simulink model "xaui_loop_delay"  (Simulink 7.0)
settings: Solver=ode45  StartTime=0.0  StopTime=100  RelTol=1e-3
undefined symbols (not defined in the file): iBOB
libraries: xbsIndex_r4 x16, xps_library x11, isi_correlator_lib x4
settings Model: Creator=wjm  LastModifiedBy=wjm

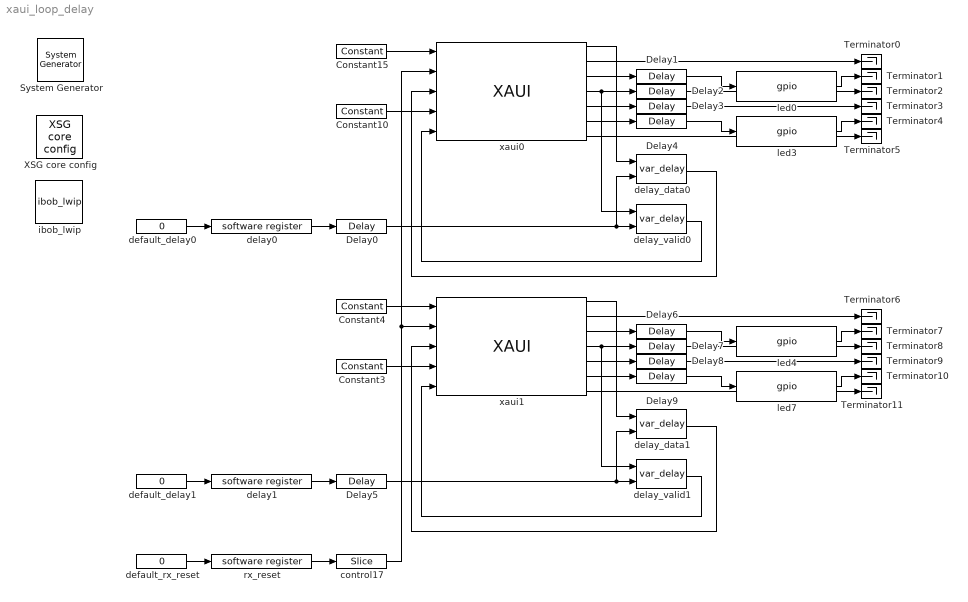
== system xaui_loop_delay ==
  " System Generator" : xbsIndex_r4/ System Generator  Tag=genX  SystemSampleTime=-1  xilinxfamily=virtex2p  part=xc2vp50  speed=-7  package=ff1152  synthesis_tool=XST  clock_wrapper=Clock Enables  directory=./xaui_loop_delay/sysgen  testbench=off  simulink_period=1  sysclk_period=5  dcm_input_clock_period=100  incr_netlist=off  trim_vbits=Everywhere in SubSystem  dbl_ovrd=According to Block Masks  core_generation=According to Block Masks  run_coregen=off  deprecated_control=off  eval_field=0  block_type=sysgen
      settings: block_version=10.1.1
  Constant10 : xbsIndex_r4/Constant  arith_type=Unsigned  const=0  n_bits=8  bin_pt=0  explicit_period=on  period=1  equ=P=C  opselect=C  inp2=PCIN>>17  opr=+  inp1=P  carry=CIN  dbl_ovrd=off  block_type=constant
      settings: block_version=10.1.1
  Constant15 : xbsIndex_r4/Constant  arith_type=Boolean  const=1  n_bits=1  bin_pt=0  explicit_period=on  period=1  equ=P=C  opselect=C  inp2=PCIN>>17  opr=+  inp1=P  carry=CIN  dbl_ovrd=off  block_type=constant
      settings: block_version=10.1.1
  Constant3 : xbsIndex_r4/Constant  arith_type=Unsigned  const=0  n_bits=8  bin_pt=0  explicit_period=on  period=1  equ=P=C  opselect=C  inp2=PCIN>>17  opr=+  inp1=P  carry=CIN  dbl_ovrd=off  block_type=constant
      settings: block_version=10.1.1
  Constant4 : xbsIndex_r4/Constant  arith_type=Boolean  const=1  n_bits=1  bin_pt=0  explicit_period=on  period=1  equ=P=C  opselect=C  inp2=PCIN>>17  opr=+  inp1=P  carry=CIN  dbl_ovrd=off  block_type=constant
      settings: block_version=10.1.1
  Delay{0..9} (10 alike) : xbsIndex_r4/Delay  en=off  latency=1  dbl_ovrd=off  reg_retiming=off  block_type=delay
  Terminator{0..11} (12 alike) : Terminator
  XSG core config : xps_library/XSG core config  Tag=xps:xsg  SystemSampleTime=-1  hw_sys=iBOB  ibob_linux=off  clk_src=sys_clk2x  iBOB_clk_src=sys_clk2x  BEE2_ctrl_clk_src=sys_clk  BEE2_usr_clk_src=sys_clk  ROACH_clk_src=adc0_clk  CORR_clk_src=sys_clk  gpio_clk_io_group=iBOB:sma  gpio_clk_bit_index=0  clk_rate=200  sample_period=1  synthesis_tool=XST  mpc_type=powerpc405
  control17 : xbsIndex_r4/Slice  nbits=1  boolean_output=on  mode=Lower Bit Location + Width  bit1=0  base1=MSB of Input  bit0=0  base0=LSB of Input  dbl_ovrd=off  block_type=slice
      settings: infoedit="Extracts a given range of bits from each input sample and presents it at the output.  The output type is ordinarily unsigned with binary point at zero, but can be Boolean when the slice is one bit wide.<P><P>Hardware notes: In hardware this block costs nothing."  block_version=10.1.3
  default_delay0 : Constant  Value=0  OutDataType=sfix(16)  OutScaling=2^0  SampleTime=1
  default_delay1 : Constant  Value=0  OutDataType=sfix(16)  OutScaling=2^0  SampleTime=1
  default_rx_reset : Constant  Value=0  OutDataType=sfix(16)  OutScaling=2^0  SampleTime=1
  delay0 : xps_library/software register  Tag=xps:sw_reg  SystemSampleTime=-1  io_dir=From Processor  arith_type=Unsigned  bitwidth=32  bin_pt=0  sample_period=1  gw_name=xaui_loop_delay_delay0_user_data_out
      link override xaui_loop_delay_delay0_user_data_out: arith_type=Unsigned  n_bits=32  bin_pt=0  period=1
  delay1 : xps_library/software register  Tag=xps:sw_reg  SystemSampleTime=-1  io_dir=From Processor  arith_type=Unsigned  bitwidth=32  bin_pt=0  sample_period=1  gw_name=xaui_loop_delay_delay1_user_data_out
      link override xaui_loop_delay_delay1_user_data_out: arith_type=Unsigned  n_bits=32  bin_pt=0  period=1
  delay_data0 : isi_correlator_lib/var_delay  SystemSampleTime=-1
  delay_data1 : isi_correlator_lib/var_delay  SystemSampleTime=-1
  delay_valid0 : isi_correlator_lib/var_delay  SystemSampleTime=-1
  delay_valid1 : isi_correlator_lib/var_delay  SystemSampleTime=-1
  ibob_lwip : xps_library/ibob_lwip  SystemSampleTime=-1
      link override macbits/convert: arith_type=Unsigned  n_bits=32  bin_pt=0
      link override machdr/xaui_loop_delay_ibob_lwip_machdr_gateway: arith_type=Unsigned  n_bits=20  bin_pt=0  period=sample_period
  led0 : xps_library/gpio  Tag=xps:gpio  SystemSampleTime=-1  io_group=iBOB:led  io_dir=out  arith_type=Boolean  bitwidth=1  bin_pt=0  bit_index=1  sample_period=1  use_single_ended=off  use_ddr=off  reg_iob=on  reg_clk_phase=0  termination=None
      link override convert: arith_type=Boolean  n_bits=1  bin_pt=0
  led3 : xps_library/gpio  Tag=xps:gpio  SystemSampleTime=-1  io_group=iBOB:led  io_dir=out  arith_type=Boolean  bitwidth=1  bin_pt=0  bit_index=2  sample_period=1  use_single_ended=off  use_ddr=off  reg_iob=on  reg_clk_phase=0  termination=None
      link override convert: arith_type=Boolean  n_bits=1  bin_pt=0
  led4 : xps_library/gpio  Tag=xps:gpio  SystemSampleTime=-1  io_group=iBOB:led  io_dir=out  arith_type=Boolean  bitwidth=1  bin_pt=0  bit_index=3  sample_period=1  use_single_ended=off  use_ddr=off  reg_iob=on  reg_clk_phase=0  termination=None
      link override convert: arith_type=Boolean  n_bits=1  bin_pt=0
  led7 : xps_library/gpio  Tag=xps:gpio  SystemSampleTime=-1  io_group=iBOB:led  io_dir=out  arith_type=Boolean  bitwidth=1  bin_pt=0  bit_index=4  sample_period=1  use_single_ended=off  use_ddr=off  reg_iob=on  reg_clk_phase=0  termination=None
      link override convert: arith_type=Boolean  n_bits=1  bin_pt=0
  rx_reset : xps_library/software register  Tag=xps:sw_reg  SystemSampleTime=-1  io_dir=From Processor  arith_type=Unsigned  bitwidth=32  bin_pt=0  sample_period=1  gw_name=xaui_loop_delay_rx_reset_user_data_out
      link override xaui_loop_delay_rx_reset_user_data_out: arith_type=Unsigned  n_bits=32  bin_pt=0  period=1
  xaui0 : xps_library/XAUI  Tag=xps:xaui  SystemSampleTime=-1  demux=2  port=iBOB:0  open_phy=on  show_param=off  pre_emph=3  swing=800
      link override convert_tx_data: n_bits=32
      link override convert_tx_outofband: n_bits=4
      link override isi_correlator_xaui0_rx_data: n_bits=32
      link override isi_correlator_xaui0_rx_outofband: n_bits=4
      link override xaui_loop_delay_xaui0_rx_data: n_bits=32
      link override xaui_loop_delay_xaui0_rx_outofband: n_bits=4
  xaui1 : xps_library/XAUI  Tag=xps:xaui  SystemSampleTime=-1  demux=2  port=iBOB:1  open_phy=on  show_param=off  pre_emph=3  swing=800
      link override convert_tx_data: n_bits=32
      link override convert_tx_outofband: n_bits=4
      link override isi_correlator_xaui0_rx_data: n_bits=32
      link override isi_correlator_xaui0_rx_outofband: n_bits=4
      link override xaui_loop_delay_xaui1_rx_data: n_bits=32
      link override xaui_loop_delay_xaui1_rx_outofband: n_bits=4
  wires:
  xaui0/2 -> Terminator0/1
  Constant15/1 -> xaui0/1
  xaui0/7 -> Terminator5/1
  Constant10/1 -> xaui0/4
  xaui0/4 -> delay_valid0/1, Delay2/1
  xaui0/3 -> Delay1/1
  xaui0/5 -> Delay3/1
  xaui0/6 -> Delay4/1
  led0/1 -> Terminator1/1
  led3/1 -> Terminator4/1
  default_delay0/1 -> delay0/1
  xaui0/1 -> delay_data0/1
  delay_data0/1 -> xaui0/3
  delay_valid0/1 -> xaui0/5
  delay0/1 -> Delay0/1
  Delay0/1 -> delay_valid0/2, delay_data0/2
  Delay1/1 -> led0/1
  Delay2/1 -> Terminator2/1
  Delay3/1 -> Terminator3/1
  Delay4/1 -> led3/1
  xaui1/2 -> Terminator6/1
  Constant4/1 -> xaui1/1
  xaui1/7 -> Terminator11/1
  Constant3/1 -> xaui1/4
  xaui1/4 -> delay_valid1/1, Delay7/1
  xaui1/3 -> Delay6/1
  xaui1/5 -> Delay8/1
  xaui1/6 -> Delay9/1
  led4/1 -> Terminator7/1
  led7/1 -> Terminator10/1
  default_delay1/1 -> delay1/1
  xaui1/1 -> delay_data1/1
  delay_data1/1 -> xaui1/3
  delay_valid1/1 -> xaui1/5
  delay1/1 -> Delay5/1
  Delay5/1 -> delay_valid1/2, delay_data1/2
  Delay6/1 -> led4/1
  Delay7/1 -> Terminator8/1
  Delay8/1 -> Terminator9/1
  Delay9/1 -> led7/1
  default_rx_reset/1 -> rx_reset/1
  rx_reset/1 -> control17/1
  control17/1 -> xaui0/2, xaui1/2
